simulink model "Sam1"  (R2018b)
settings: Solver=FixedStepAuto  StartTime=0.0  StopTime=10.0  RelTol=1e-3
libraries: simulink x1
settings Model: Creator=Amir  LastModifiedBy=Amir

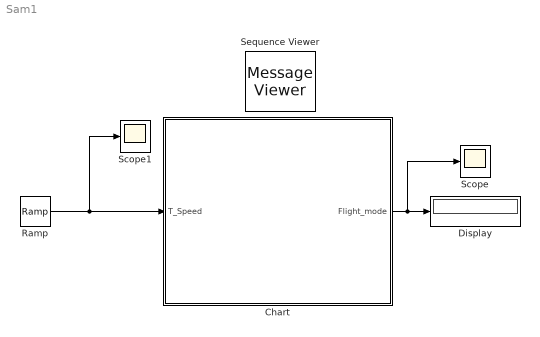
== system Sam1 ==
  Chart : Stateflow chart  TreatAsAtomicUnit=on
  Display : Display
  Ramp : simulink/Sources/Ramp  slope=-2  start=0  InitialOutput=55
  Scope : Scope
  Scope1 : Scope
  Sequence Viewer : MessageViewer
  wires:
  Chart/1(Flight_mode) -> Scope/1, Display/1
  Ramp/1 -> Scope1/1, Chart/1(T_Speed)

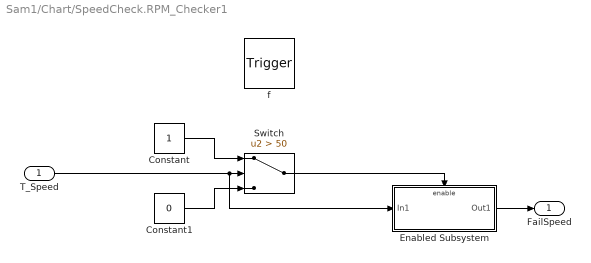
== system Sam1/Chart/SpeedCheck.RPM_Checker1 ==
  T_Speed : Inport
  f : TriggerPort  TriggerType=function-call  VariantControl=(inherit)
      settings: CopyFcn=Stateflow.SLINSF.SimulinkMan.removeBlockPreDeleteFcn  PreDeleteFcn=Stateflow.SLINSF.SimulinkMan.unsafePredeleteFcn
  Constant : Constant
  Constant1 : Constant  Value=0
  Enabled Subsystem : Subsystem  TreatAsAtomicUnit=on
  Switch : Switch  Criteria=u2 > Threshold  Threshold=50
  FailSpeed : Outport
  wires:
  Constant1/1 -> Switch/3
  Switch/1 -> Enabled Subsystem/Enable
  Constant/1 -> Switch/1
  T_Speed/1 -> Enabled Subsystem/1(In1), Switch/2
  Enabled Subsystem/1(Out1) -> FailSpeed/1

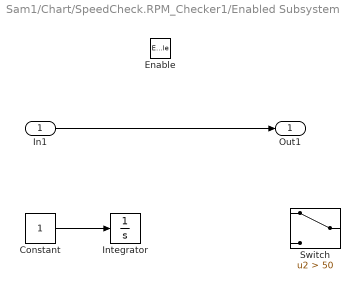
== system Sam1/Chart/SpeedCheck.RPM_Checker1/Enabled Subsystem ==
  In1 : Inport
  Enable : EnablePort  StatesWhenEnabling=reset
  Constant : Constant
  Integrator : Integrator
  Switch : Switch  Criteria=u2 > Threshold  Threshold=50
  Out1 : Outport
  wires:
  In1/1 -> Out1/1
  Constant/1 -> Integrator/1

== stateflow chart Sam1/Chart ==
  state Motor [parallel]
    settings: executionOrder=2
    state RPM
      if T_Speed<50
      Fail_Speed=1;
      else
      Flight_mode=0;
      Fail_Speed=0;
      end
    (default) -> RPM
  state SpeedCheck [parallel]
    settings: executionOrder=1
    state TAS
      FailSpeed = RPM_Checker1(T_Speed)
      if T_Speed<50
      Fail_Speed=1;
      else
      Flight_mode=0;
      Fail_Speed=0;
      end
    state TAS1
      if T_Speed<50
      Fail_Speed=1;
      else
      Flight_mode=0;
      Fail_Speed=0;
      end
    state FailSpeed = RPM_Checker1(T_Speed) [function]
    (default) -> SpeedCheck.TAS
    TAS1 -> SpeedCheck.TAS : [after(2)]
    SpeedCheck.TAS -> TAS1
  state SpeedCheck1 [parallel]
    settings: executionOrder=3
    state TAS
      if T_Speed<50
      Fail_Speed=1;
      else
      Flight_mode=0;
      Fail_Speed=0;
      end
    (default) -> SpeedCheck1.TAS
  state SpeedCheck2 [parallel]
    settings: executionOrder=4
    state TAS
      if T_Speed<50
      Fail_Speed=1;
      else
      Flight_mode=0;
      Fail_Speed=0;
      end
    (default) -> SpeedCheck2.TAS
  state SpeedCheck4 [parallel]
    settings: executionOrder=6
    state TAS
      if T_Speed<50
      Fail_Speed=1;
      else
      Flight_mode=0;
      Fail_Speed=0;
      end
    (default) -> SpeedCheck4.TAS
  state SpeedCheck3 [parallel]
    settings: executionOrder=5
    state TAS
      if T_Speed<50
      Fail_Speed=1;
      else
      Flight_mode=0;
      Fail_Speed=0;
      end
    (default) -> SpeedCheck3.TAS
  data: T_Speed function_input; FailSpeed function_output; T_Speed input; Flight_mode output; Fail_Speed local
